simulink model "Simulateur_V1_eq06 (1)"  (R2025b)
settings: Solver=FixedStepAuto  StartTime=0.0  StopTime=30  FixedStep=1e-5  RelTol=1e-3
model workspace (MAT data in the model file):
  B = 0.1128
  Br = 1.2
  D = 0.002
  E = 17000000000
  Filt = 0.09
  GainAmpliPuissance = 1.86
  L = 0.244
  N = 66
  R = 0.016
  b = 0.43454
  cap = -0.111
  dens = 1850
  freq = 0.00204081632653
  h = 0.0015
  l = 0.07
  m = 0.05
  m_supp = 0.03
  q = 0.135
  r = 0.0203
  temp_add = 6
settings Model: Creator=jeann
settings RTWCC: GPUComputeCapability=3.5

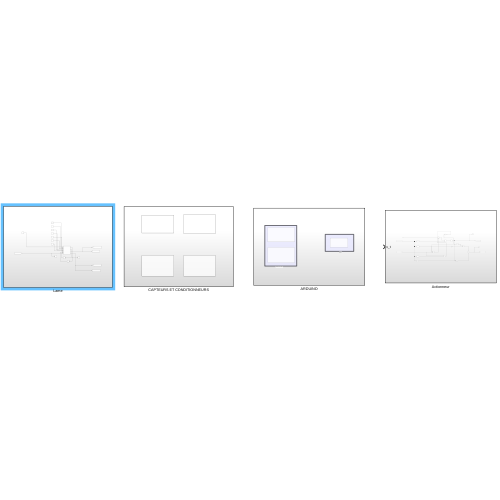
[thumbnail: Simulink's stored preview of the top-level diagram]
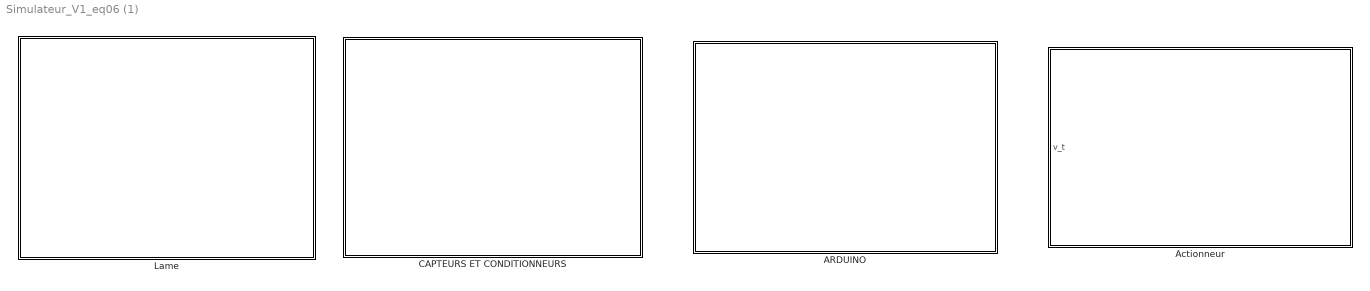
== system Simulateur_V1_eq06 (1) ==
  ARDUINO : Subsystem
  Actionneur : Subsystem
  CAPTEURS ET CONDITIONNEURS : Subsystem
  Lame : Subsystem

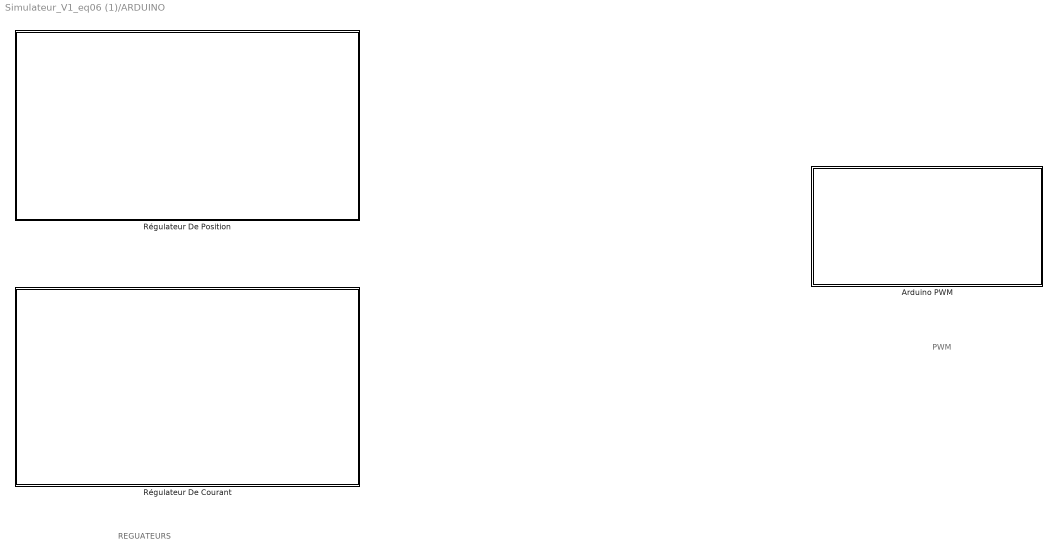
== system Simulateur_V1_eq06 (1)/ARDUINO ==
  note: REGUATEURS
  note: PWM
  Arduino PWM : Subsystem
  Régulateur De Courant : Subsystem
  Régulateur De Position : Subsystem

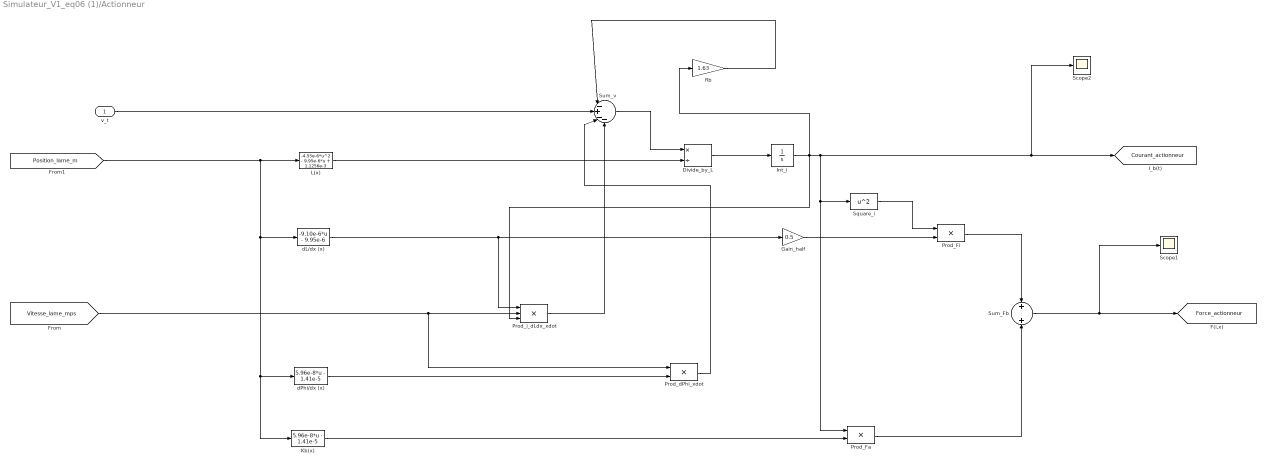
== system Simulateur_V1_eq06 (1)/Actionneur ==
  v_t : Inport
  Divide_by_L : Product  Inputs=*/
  Gain_half : Gain  Gain=0.5
  Int_i : Integrator
  Kb(x) : Fcn  Expr=5.96e-8*u - 1.41e-5
  L(x) : Fcn  Expr=-4.55e-6*u^2 - 9.95e-6*u + 1.1256e-3
  Prod_Fa : Product
  Prod_Fi : Product
  Prod_dPhi_xdot : Product
  Prod_i_dLdx_xdot : Product  Inputs=3
  Rb : Gain  Gain=1.63
  Scope1 : Scope
      settings: DataLoggingVariableName=ScopeData5
  Scope2 : Scope
      settings: DataLoggingVariableName=ScopeData9
  Square_i : Math  Operator=square
  Sum_Fb : Sum
  Sum_v : Sum  Inputs=|-+--
  dL/dx (x) : Fcn  Expr=-9.10e-6*u - 9.95e-6
  dPhi/dx (x) : Fcn  Expr=5.96e-8*u - 1.41e-5
  tag scope: Courant_actionneur=global, Force_actionneur=global
  wires:
  dL/dx (x)/1 -> Gain_half/1, Prod_i_dLdx_xdot/1
  Prod_Fi/1 -> Sum_Fb/1
  Sum_Fb/1 -> Scope1/1, [Force_actionneur]
  Rb/1 -> Sum_v/1
  Prod_Fa/1 -> Sum_Fb/2
  v_t/1 -> Sum_v/2
  Prod_i_dLdx_xdot/1 -> Sum_v/4
  L(x)/1 -> Divide_by_L/2
  Square_i/1 -> Prod_Fi/1
  Prod_dPhi_xdot/1 -> Sum_v/3
  Gain_half/1 -> Prod_Fi/2
  dPhi/dx (x)/1 -> Prod_dPhi_xdot/2
  Divide_by_L/1 -> Int_i/1
  Int_i/1 -> Prod_i_dLdx_xdot/3, Scope2/1, [Courant_actionneur], Square_i/1, Prod_Fa/1, Rb/1
  Sum_v/1 -> Divide_by_L/1
  [Vitesse_lame_mps] -> Prod_dPhi_xdot/1, Prod_i_dLdx_xdot/2
  Kb(x)/1 -> Prod_Fa/2
  [Position_lame_m] -> dL/dx (x)/1, Kb(x)/1, dPhi/dx (x)/1, L(x)/1

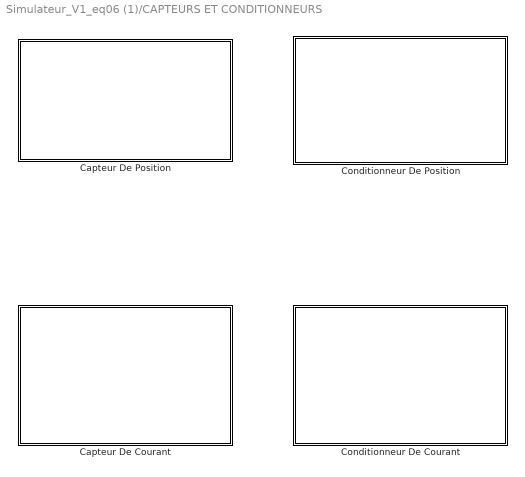
== system Simulateur_V1_eq06 (1)/CAPTEURS ET CONDITIONNEURS ==
  Capteur De Courant : Subsystem
  "Capteur De Position " : Subsystem
  Conditionneur De Courant : Subsystem
  Conditionneur De Position : Subsystem

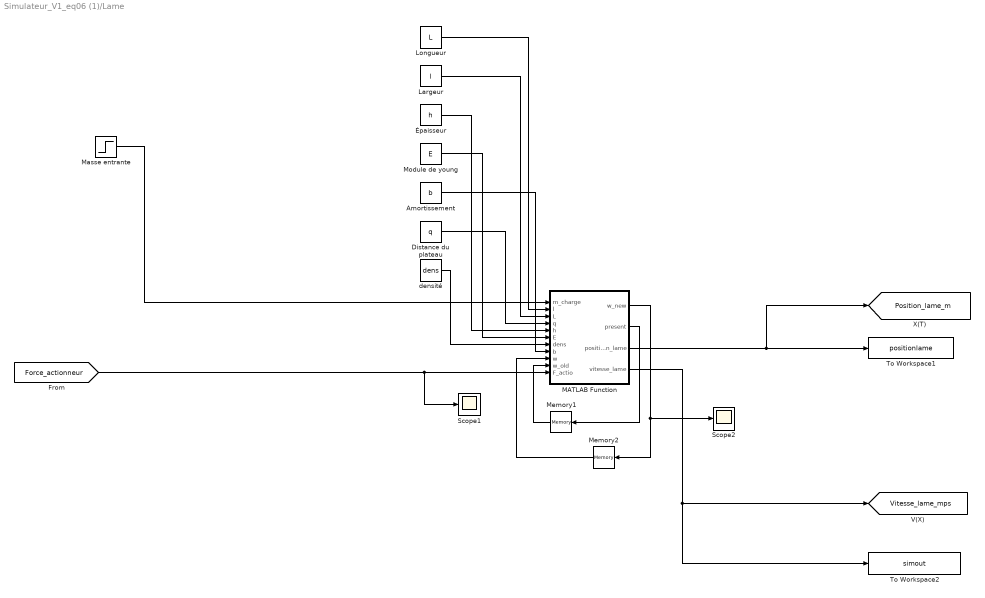
== system Simulateur_V1_eq06 (1)/Lame ==
  Amortissement : Constant  Value=b
  Distance du plateau : Constant  Value=q
  Largeur : Constant  Value=l
  Longueur : Constant  Value=L
  MATLAB Function : MATLAB Function  TreatAsAtomicUnit=on
  Masse entrante : Step  After=m  SampleTime=3
  Memory1 : Memory  InitialCondition=zeros(12,1)
  Memory2 : Memory  InitialCondition=zeros(12,1)  StateName=matrix
  Module de young : Constant  Value=E
  Scope1 : Scope
      settings: ActiveDisplayYMinimum=-0.06178  ActiveDisplayYMaximum=0.55605  DataLoggingVariableName=ScopeData10
  Scope2 : Scope
      settings: ActiveDisplayYMinimum=-0.01789  ActiveDisplayYMaximum=0.00274
  To Workspace1 : ToWorkspace  VariableName=positionlame  SaveFormat=Timeseries  SampleTime=-1
  To Workspace2 : ToWorkspace  VariableName=simout  SaveFormat=Timeseries  SampleTime=-1
  densité : Constant  Value=dens
  Épaisseur : Constant  Value=h
  tag scope: Position_lame_m=global, Vitesse_lame_mps=global
  wires:
  [Force_actionneur] -> Scope1/1, MATLAB Function/11(F_actio)
  Longueur/1 -> MATLAB Function/2(l)
  MATLAB Function/1(w_new) -> Memory2/1, Scope2/1
  Memory2/1 -> MATLAB Function/9(w)
  MATLAB Function/2(present) -> Memory1/1
  Memory1/1 -> MATLAB Function/10(w_old)
  Largeur/1 -> MATLAB Function/3(L)
  Épaisseur/1 -> MATLAB Function/5(h)
  Module de young/1 -> MATLAB Function/6(E)
  Amortissement/1 -> MATLAB Function/8(b)
  Distance du plateau/1 -> MATLAB Function/4(q)
  densité/1 -> MATLAB Function/7(dens)
  Masse entrante/1 -> MATLAB Function/1(m_charge)
  MATLAB Function/3(position_lame) -> [Position_lame_m], To Workspace1/1
  MATLAB Function/4(vitesse_lame) -> [Vitesse_lame_mps], To Workspace2/1

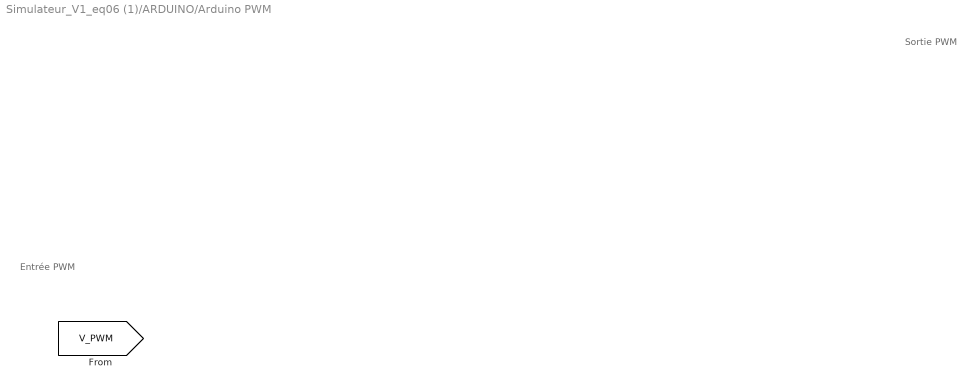
== system Simulateur_V1_eq06 (1)/ARDUINO/Arduino PWM ==
  note: Entrée PWM
  note: Sortie PWM

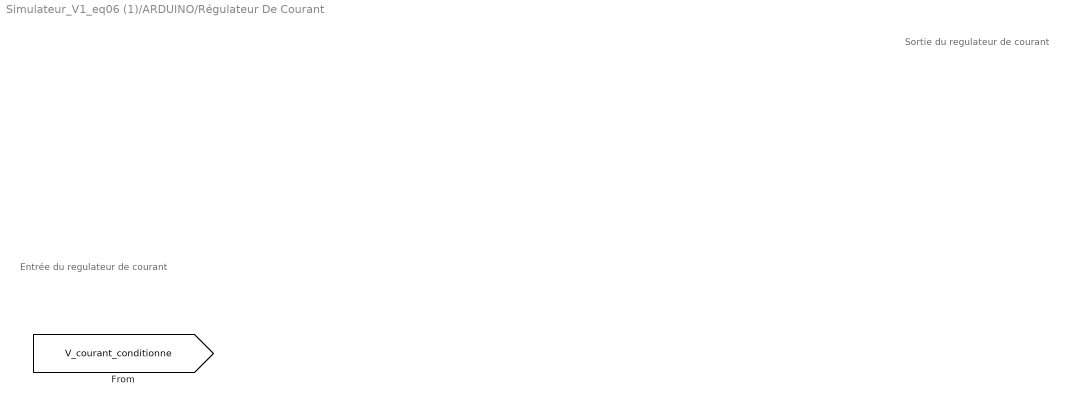
== system Simulateur_V1_eq06 (1)/ARDUINO/Régulateur De Courant ==
  note: Sortie du regulateur de courant
  note: Entrée du regulateur de courant

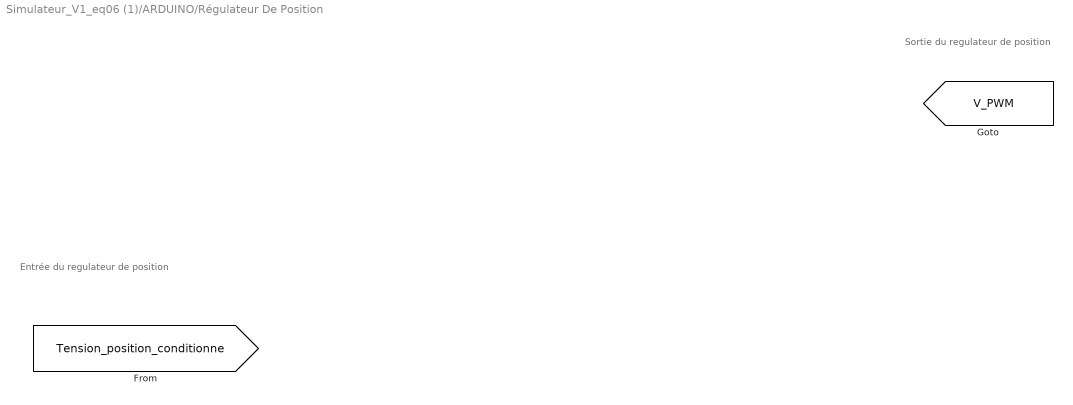
== system Simulateur_V1_eq06 (1)/ARDUINO/Régulateur De Position ==
  note: Sortie du regulateur de position
  note: Entrée du regulateur de position
  tag scope: V_PWM=global

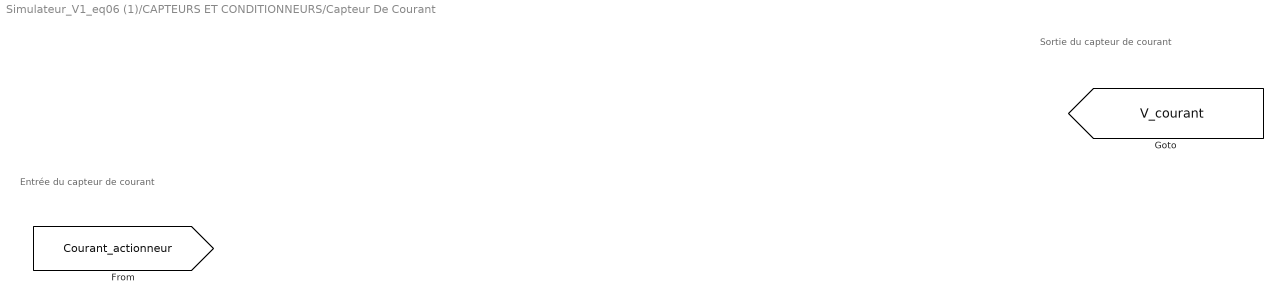
== system Simulateur_V1_eq06 (1)/CAPTEURS ET CONDITIONNEURS/Capteur De Courant ==
  note: Sortie du capteur de courant
  note: Entrée du capteur de courant
  tag scope: V_courant=global

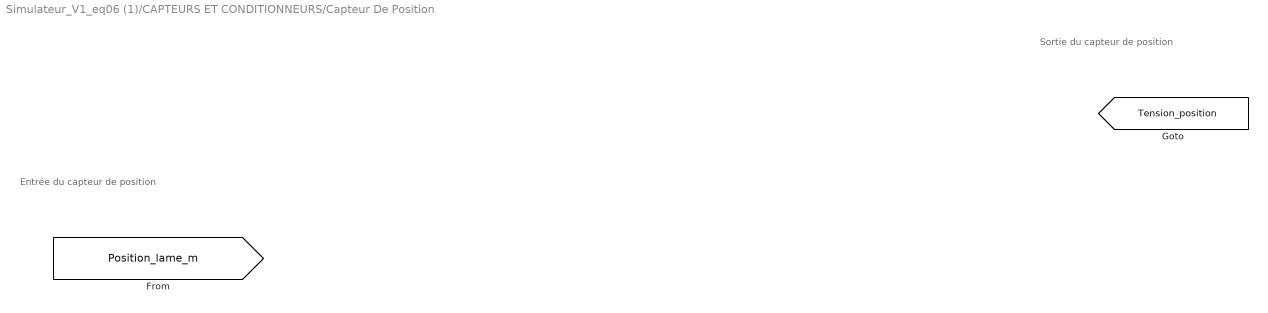
== system Simulateur_V1_eq06 (1)/CAPTEURS ET CONDITIONNEURS/Capteur De Position  ==
  note: Entrée du capteur de position
  note: Sortie du capteur de position
  tag scope: Tension_position=global

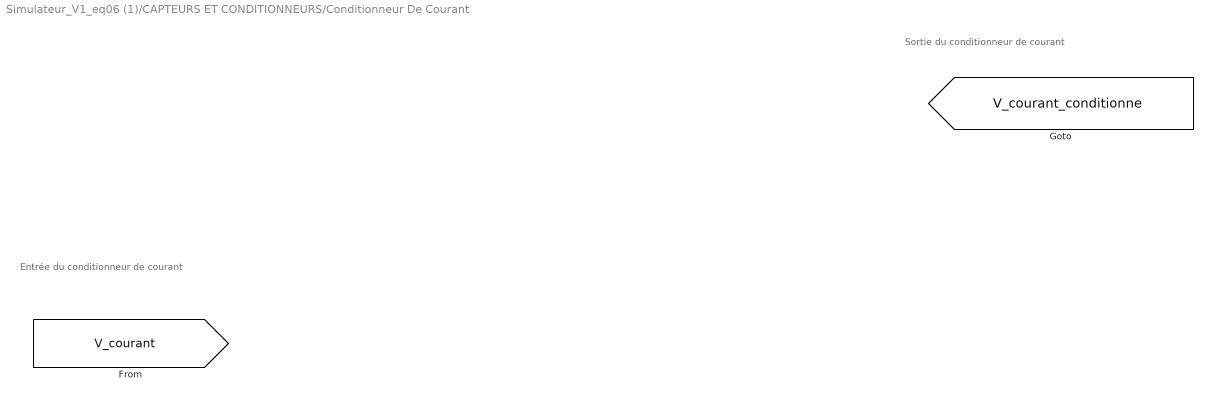
== system Simulateur_V1_eq06 (1)/CAPTEURS ET CONDITIONNEURS/Conditionneur De Courant ==
  note: Sortie du conditionneur de courant
  note: Entrée du conditionneur de courant
  tag scope: V_courant_conditionne=global

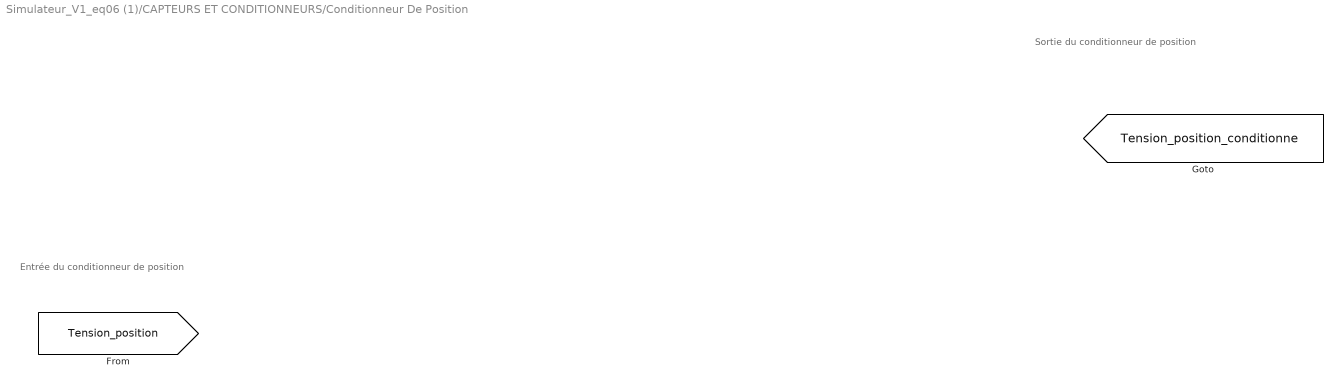
== system Simulateur_V1_eq06 (1)/CAPTEURS ET CONDITIONNEURS/Conditionneur De Position ==
  note: Sortie du conditionneur de position
  note: Entrée du conditionneur de position
  tag scope: Tension_position_conditionne=global

== matlab function Simulateur_V1_eq06 (1)/Lame/MATLAB Function ==
  data: m_charge input; w_new output; l input; L input; q input; h input; E input; dens input; b input; w input; w_old input; present output; position_lame output; F_actio input; vitesse_lame output
function [w_new, present, position_lame, vitesse_lame] = fcn(m_charge, l, L, q, h, E, dens, b, w, w_old, F_actio)

% =========================
% Paramètres de la poutre
% =========================
J = L*h^3/12;          % Moment quadratique de la section [m^4]
mu = dens*L*h;         % Masse linéique [kg/m]

% =========================
% Paramètres physiques
% =========================
m_lame   = mu*l;       % Masse totale de la lame [kg]
m_aimant = 9.3e-3;     % Masse de l'aimant [kg]
g = -9.8;              % Gravité [m/s^2]
dt = 1e-5;             % Pas de temps [s]

% =========================
% Discrétisation spatiale
% =========================
nx = 10;               % Nombre de noeuds internes utiles
dx = l/(nx-1);         % Pas spatial [m]

% Position discrète de la masse / force appliquée
q_i = 2 + round(q/dx);

% Ajout de 2 noeuds fantômes pour les conditions limites
nx = nx + 2;

% =========================
% Vecteur des forces
% =========================
F = zeros(nx,1);
F(end) = g*m_aimant;              % Poids de l'aimant au bout
F(q_i) = g*m_charge + F_actio;     % Poids de la pièce + force actionneur

% =========================
% Coefficients de calcul
% =========================
coeff1  = -E*J*dt^2/(mu*dx^4);
coeff2  = -(dt^2/mu)*(-2*mu/dt^2 + b/dt);
coeff3  = -(dt^2/mu)*( mu/dt^2 - b/dt);
coeff_F = dt^2/(mu*dx);

% =========================
% Initialisation
% =========================
w_new = zeros(nx,1);

% =========================
% Mise à jour de la déformation
% =========================
i = 3:nx-2;

w_new(i) = coeff1 * ( w(i+2) - 4*w(i+1) + 6*w(i) - 4*w(i-1) + w(i-2) ) ...
         + coeff2 * w(i) ...
         + coeff3 * w_old(i) ...
         + coeff_F * F(i);

% =========================
% Conditions limites
% =========================
w_new(1:2) = 0;    % Encastrement : déplacement et pente nuls

% Extrémité libre : dérivées 2e et 3e nulles
w_new(end-1) = 2*w_new(end-2) - w_new(end-3);
w_new(end)   = 2*w_new(end-1) - w_new(end-2);

% =========================
% Sorties
% =========================
present = w;                            % Etat actuel pour mémoire
position_lame = w_new(end);             % Position au bout de la lame [m]
vitesse_lame  = (w_new(end) - w(end))/dt; % Vitesse au bout [m/s]


end
